simulink model "asbhl20_GuidanceApp"  (R2016b)
settings: Solver=FixedStepDiscrete  StartTime=0.0  StopTime=10.0  FixedStep=1/60  RelTol=1e-3
values from neighbouring files (symbols this model uses):
  Aimpoint = 500    [asbhl20_GuidanceAppData.mat]
  alpha0 = 0.114253174362    [asbhl20_GuidanceAppData.mat]
  fitdata =     [asbhl20_GuidanceAppData.mat]
  glideslope_offset = 20    [asbhl20_GuidanceAppData.mat]
  heading0 = 117    [asbhl20_GuidanceAppData.mat]
  hglide = [2 2.4375 2.875 3.3125 3.75 4.1875 4.625 5.0625 5.5 5.9375 6.375 6.8125 ... (668 elements, 668x1)]    [asbhl20_GuidanceAppData.mat]
  Xglide = [-675 -650 -625 -600 -575 -550 -525 -500 -475 -450 -425 -400 ... (668 elements, 668x1)]    [asbhl20_GuidanceAppData.mat]
undefined symbols (not defined in the file or in its folder): DiscIntNeverNeededParam, Earth, Tc, WGS84
libraries: asbhl20scdexblks x4, simulink x2, aerolibtransform2 x1, aerolibobsolete x1, aerolibconvert2 x1
Description:
  | HL-20 guidance control system module
settings Model: FPTRunName=Active  ExtModeAutoUpdateStatusClock=off  Creator=The MathWorks, Inc.  LastModifiedBy=The MathWorks, Inc.
settings DataIOCC: SaveFormat=Array  SaveOutput=off  SaveTime=off
settings OptimizationCC: BlockReduction=off  DefaultParameterBehavior=Inlined  OptimizeBlockIOStorage=off  BufferReuse=off  GlobalBufferReuse=off  ExpressionFolding=off  ExpressionDepthLimit=2147483647  LocalBlockOutputs=off  InitFltsAndDblsToZero=on  LifeSpan=inf
settings DebuggingCC: AlgebraicLoopMsg=none  UnderspecifiedInitializationDetection=Classic  MultiTaskCondExecSysMsg=none  FcnCallInpInsideContextMsg=warning  UnconnectedInputMsg=none  UnconnectedOutputMsg=none  UnconnectedLineMsg=none  UniqueDataStoreMsg=error  AllowSymbolicDim=off  StateNameClashWarn=warning  StrictBusMsg=ErrorOnBusTreatedAsVector  SFUnexpectedBacktrackingDiag=warning  SFNoUnconditionalDefaultTransitionDiag=warning  SFExecutionAtInitializationDiag=none
settings HardwareCC: ProdBitPerPointer=32  ProdBitPerSizeT=32  ProdBitPerPtrDiffT=32  ProdLargestAtomicFloat=None  ProdIntDivRoundTo=Undefined  ProdEndianess=Unspecified  ProdWordSize=32  ProdHWDeviceType=32-bit Generic
settings ModelReferenceCC: UpdateModelReferenceTargets=AssumeUpToDate  CheckModelReferenceTargetMessage=none  ModelReferencePassRootInputsByReference=off  PropagateSignalLabelsOutOfModel=off
settings CodeAppCC: MaxIdLength=63
settings GRTTargetCC: TargetLangStandard=C89/C90 (ANSI)  GeneratePreprocessorConditionals=Disable all  CombineOutputUpdateFcns=off  GRTInterface=on
settings ConfigComp: CovMetricSettings=dw  CovHtmlReporting=on  CovSaveCumulativeToWorkspaceVar=on  CovSaveSingleToWorkspaceVar=on  CovExternalEMLEnable=off  CovSFcnEnable=off

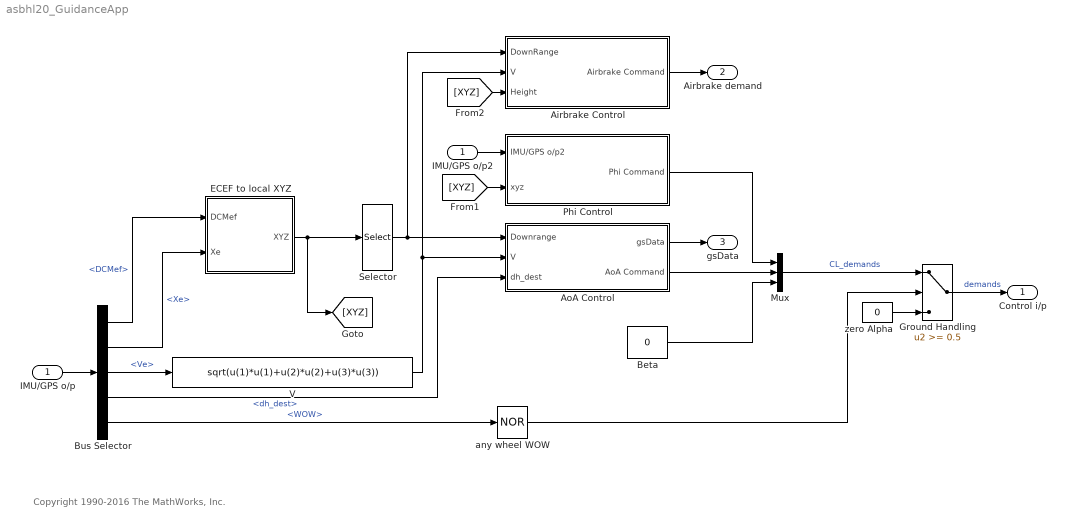
== system asbhl20_GuidanceApp ==
  note: Copyright 1990-2016 The MathWorks, Inc.
  IMU/GPS o/p : Inport  OutDataTypeStr=Bus: GuidanceBus
  Airbrake Control : Subsystem
  AoA Control : Subsystem
  Beta : Constant  Value=0  OutDataTypeStr=float('double')  SampleTime=Tc
  Bus Selector : BusSelector  OutputSignals=DCMef,Xe,Ve,dh_dest,WOW
  ECEF to local XYZ : Subsystem
  Ground Handling : Switch  Threshold=0.5  SaturateOnIntegerOverflow=on  InputSameDT=on
  IMU/GPS o/p2 : InportShadow  OutDataTypeStr=Bus: GuidanceBus
  Mux : Mux  Inputs=3
  Phi Control : Subsystem
  Selector : Selector  InputPortWidth=3  IndexOptions=Index vector (dialog)  Indices=1  OutputSizes=1
  V : Fcn  Expr=sqrt(u(1)*u(1)+u(2)*u(2)+u(3)*u(3))
  any wheel WOW : Logic  Operator=NOR  Inputs=1  IconShape=distinctive  AllPortsSameDT=off  OutDataTypeStr=boolean
  zero Alpha : Constant  Value=0  OutDataTypeStr=float('double')  SampleTime=Tc
  Control i/p : Outport
  Airbrake demand : Outport  Port=2
  gsData : Outport  Port=3  OutDataTypeStr=Bus: gsDataBus
  wires:
  Bus Selector/5 -> any wheel WOW/1  "<WOW>"
  any wheel WOW/1 -> Ground Handling/2
  Ground Handling/1 -> Control i/p/1  "demands"
  V/1 -> Airbrake Control/2(V), AoA Control/2(V)
  Mux/1 -> Ground Handling/1  "CL_demands"
  Bus Selector/2 -> ECEF to local XYZ/2(Xe)  "<Xe>"
  Bus Selector/3 -> V/1  "<Ve>"
  IMU/GPS o/p/1 -> Bus Selector/1
  Bus Selector/1 -> ECEF to local XYZ/1(DCMef)  "<DCMef>"
  ECEF to local XYZ/1(XYZ) -> [XYZ], Selector/1
  Selector/1 -> Airbrake Control/1(DownRange), AoA Control/1(Downrange)
  Phi Control/1(Phi Command) -> Mux/1
  IMU/GPS o/p2/1 -> Phi Control/1(IMU/GPS o/p2)
  zero Alpha/1 -> Ground Handling/3
  [XYZ] -> Phi Control/2(xyz)
  [XYZ] -> Airbrake Control/3(Height)
  Airbrake Control/1(Airbrake Command) -> Airbrake demand/1
  AoA Control/1(gsData) -> gsData/1
  AoA Control/2(AoA Command) -> Mux/2
  Bus Selector/4 -> AoA Control/3(dh_dest)  "<dh_dest>"
  Beta/1 -> Mux/3

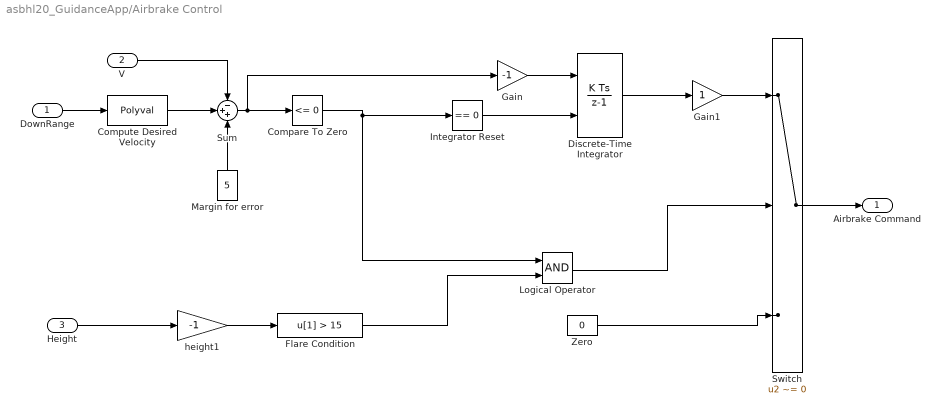
== system asbhl20_GuidanceApp/Airbrake Control ==
  DownRange : Inport
  V : Inport  Port=2
  Height : Inport  Port=3
  Compare To Zero : simulink/Logic and Bit Operations/Compare To Zero  relop=<=  OutDataTypeStr=uint8  ZeroCross=off
  Compute Desired Velocity : Polyval  Coefs=fitdata.coeff
  Discrete-Time Integrator : DiscreteIntegrator  ExternalReset=level  InitialConditionSetting=State (most efficient)  SampleTime=Tc  LimitOutput=on  UpperSaturationLimit=50  LowerSaturationLimit=-50  ICPrevOutput=DiscIntNeverNeededParam  ICPrevScaledInput=DiscIntNeverNeededParam
  Flare Condition : Fcn  Expr=u[1] > 15
  Gain : Gain  Gain=-1
  Gain1 : Gain
  Integrator Reset : simulink/Logic and Bit Operations/Compare To Zero  relop===  OutDataTypeStr=uint8  ZeroCross=off
  Logical Operator : Logic  AllPortsSameDT=off  OutDataTypeStr=boolean
  Margin for error : Constant  Value=5  OutDataTypeStr=float('double')  SampleTime=Tc
  Sum : Sum  Inputs=-++
  Switch : Switch  Criteria=u2 ~= 0
  Zero : Constant  Value=0  OutDataTypeStr=float('double')  SampleTime=Tc
  height1 : Gain  Gain=-1  SaturateOnIntegerOverflow=on  OutDataTypeStr=Inherit: Same as input  ParamDataTypeStr=Inherit: Same as input
  Airbrake Command : Outport
  wires:
  V/1 -> Sum/1
  Margin for error/1 -> Sum/3
  Gain1/1 -> Switch/1
  Logical Operator/1 -> Switch/2
  Flare Condition/1 -> Logical Operator/2
  height1/1 -> Flare Condition/1
  Height/1 -> height1/1
  Switch/1 -> Airbrake Command/1
  Zero/1 -> Switch/3
  Integrator Reset/1 -> Discrete-Time Integrator/2
  Discrete-Time Integrator/1 -> Gain1/1
  Gain/1 -> Discrete-Time Integrator/1
  Compare To Zero/1 -> Logical Operator/1, Integrator Reset/1
  Compute Desired Velocity/1 -> Sum/2
  Sum/1 -> Gain/1, Compare To Zero/1
  DownRange/1 -> Compute Desired Velocity/1

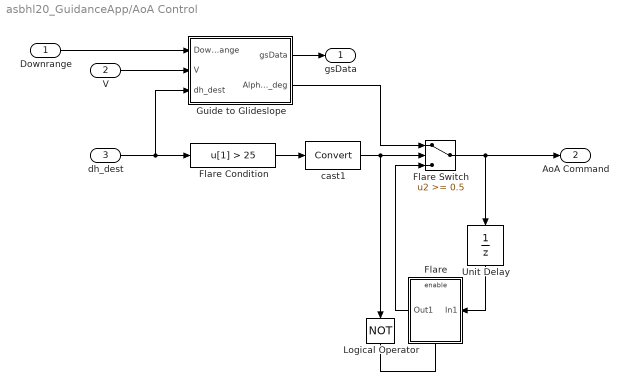
== system asbhl20_GuidanceApp/AoA Control ==
  Downrange : Inport
  V : Inport  Port=2
  dh_dest : Inport  Port=3
  Flare : Subsystem  TreatAsAtomicUnit=on
  Flare Condition : Fcn  Expr=u[1] > 25
  Flare Switch : Switch  Threshold=0.5  SaturateOnIntegerOverflow=on  InputSameDT=on
  Guide to Glideslope : Subsystem
  Logical Operator : Logic  Operator=NOT  IconShape=distinctive
  Unit Delay : UnitDelay  SampleTime=4*Tc
  cast1 : DataTypeConversion  SaturateOnIntegerOverflow=on  RndMeth=Zero
  gsData : Outport  OutDataTypeStr=Bus: gsDataBus
  AoA Command : Outport  Port=2
  wires:
  Guide to Glideslope/1(gsData) -> gsData/1
  Guide to Glideslope/2(AlphaD_deg) -> Flare Switch/1
  Logical Operator/1 -> Flare/Enable
  Flare/1(Out1) -> Flare Switch/3
  Flare Switch/1 -> Unit Delay/1, AoA Command/1
  Flare Condition/1 -> cast1/1
  cast1/1 -> Logical Operator/1, Flare Switch/2
  Unit Delay/1 -> Flare/1(In1)
  dh_dest/1 -> Flare Condition/1, Guide to Glideslope/3(dh_dest)
  Downrange/1 -> Guide to Glideslope/1(Downrange)
  V/1 -> Guide to Glideslope/2(V)

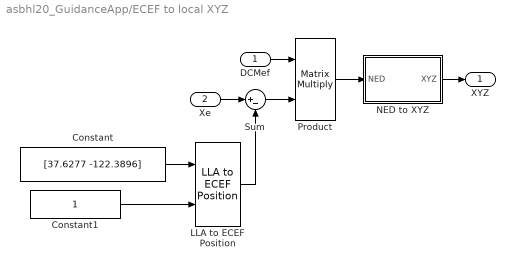
== system asbhl20_GuidanceApp/ECEF to local XYZ ==
  DCMef : Inport
  Xe : Inport  Port=2
  Constant : Constant  Value=[37.6277 -122.3896]
  Constant1 : Constant
  LLA to ECEF Position : aerolibtransform2/LLA to ECEF Position  units=Metric (MKS)  ptype=Earth (WGS84)  F=1/298.257223563  R=6378137
  NED to XYZ : Subsystem
  Product : Product  Multiplication=Matrix(*)  RndMeth=Zero
  Sum : Sum  Inputs=|+-
  XYZ : Outport
  wires:
  Sum/1 -> Product/2
  Constant1/1 -> LLA to ECEF Position/2
  Constant/1 -> LLA to ECEF Position/1
  LLA to ECEF Position/1 -> Sum/2
  Product/1 -> NED to XYZ/1(NED)
  DCMef/1 -> Product/1
  NED to XYZ/1(XYZ) -> XYZ/1
  Xe/1 -> Sum/1

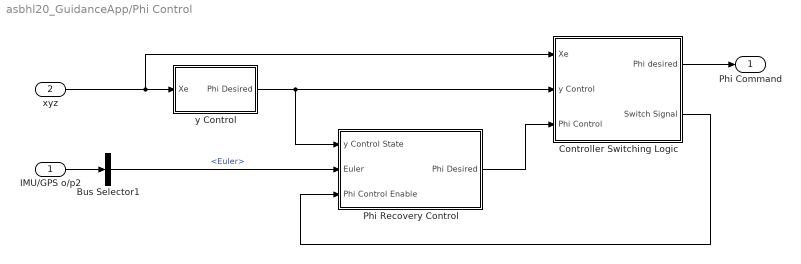
== system asbhl20_GuidanceApp/Phi Control ==
  IMU/GPS o/p2 : Inport
  xyz : Inport  Port=2
  Bus Selector1 : BusSelector  OutputSignals=Euler
  Controller Switching Logic : Subsystem
  Phi Recovery Control : Subsystem
  y Control : Subsystem
  Phi Command : Outport
  wires:
  y Control/1(Phi Desired) -> Phi Recovery Control/1(y Control State), Controller Switching Logic/2(y Control)
  Phi Recovery Control/1(Phi Desired) -> Controller Switching Logic/3(Phi Control)
  Controller Switching Logic/2(Switch Signal) -> Phi Recovery Control/3(Phi Control Enable)
  IMU/GPS o/p2/1 -> Bus Selector1/1
  Controller Switching Logic/1(Phi desired) -> Phi Command/1
  Bus Selector1/1 -> Phi Recovery Control/2(Euler)  "<Euler>"
  xyz/1 -> y Control/1(Xe), Controller Switching Logic/1(Xe)

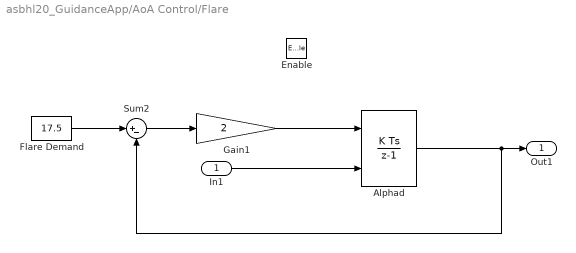
== system asbhl20_GuidanceApp/AoA Control/Flare ==
  In1 : Inport  SampleTime=Tc
  Enable : EnablePort  StatesWhenEnabling=reset
  Alphad : DiscreteIntegrator  InitialConditionSource=external  SampleTime=Tc  LimitOutput=on  UpperSaturationLimit=35  LowerSaturationLimit=-10  ICPrevOutput=DiscIntNeverNeededParam  ICPrevScaledInput=DiscIntNeverNeededParam
  Flare Demand : Constant  Value=17.5  OutDataTypeStr=float('double')
  Gain1 : Gain  Gain=2  SaturateOnIntegerOverflow=on  OutDataTypeStr=Inherit: Same as input  ParamDataTypeStr=Inherit: Same as input
  Sum2 : Sum  Inputs=|+-  SaturateOnIntegerOverflow=on  InputSameDT=on  OutDataTypeStr=Inherit: Same as first input
  Out1 : Outport
  wires:
  Alphad/1 -> Out1/1, Sum2/2
  Gain1/1 -> Alphad/1
  Sum2/1 -> Gain1/1
  Flare Demand/1 -> Sum2/1
  In1/1 -> Alphad/2

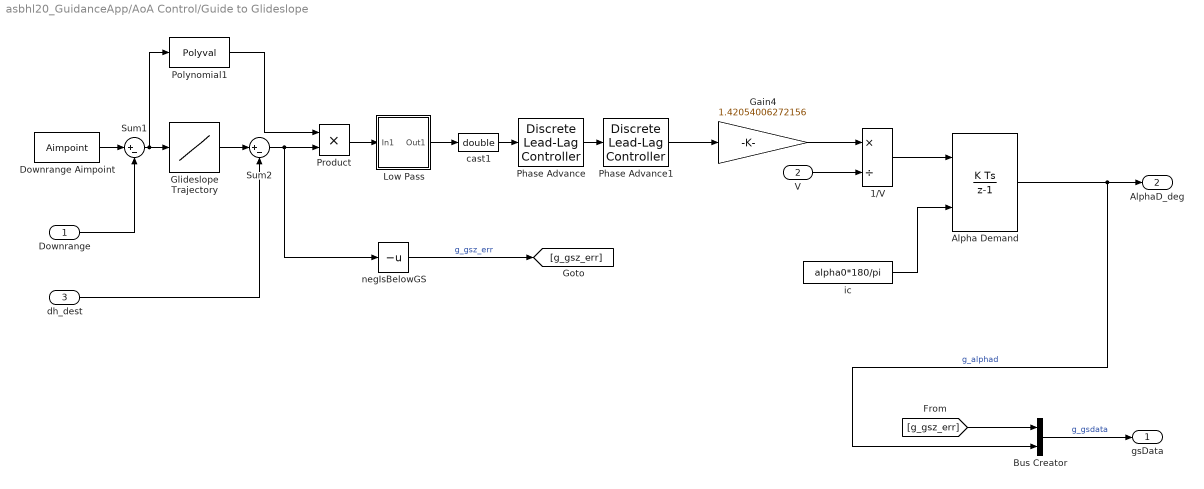
== system asbhl20_GuidanceApp/AoA Control/Guide to Glideslope ==
  Downrange : Inport
  V : Inport  Port=2
  dh_dest : Inport  Port=3
  1/V : Product  Inputs=*/  SaturateOnIntegerOverflow=on  InputSameDT=on  OutDataTypeStr=Inherit: Same as first input
  Alpha Demand : DiscreteIntegrator  InitialConditionSource=external  SampleTime=Tc  LimitOutput=on  UpperSaturationLimit=15  LowerSaturationLimit=0  ICPrevOutput=DiscIntNeverNeededParam  ICPrevScaledInput=DiscIntNeverNeededParam
  Bus Creator : BusCreator  Inputs=2  OutDataTypeStr=Bus: gsDataBus
  Downrange Aimpoint : Constant  Value=Aimpoint  OutDataTypeStr=float('double')
  Gain4 : Gain  Gain=1.42054006272156  SaturateOnIntegerOverflow=on  OutDataTypeStr=Inherit: Same as input  ParamDataTypeStr=Inherit: Same as input
  Glideslope Trajectory : Lookup_n-D  NumberOfTableDimensions=1  BreakpointsForDimension1=Xglide  Table=hglide+glideslope_offset  SaturateOnIntegerOverflow=on
  Low Pass : Subsystem
  Phase Advance : asbhl20scdexblks/Discrete Lead-Lag Controller  Zero=0.0620701951848126  Pole=16.8176549917091  Ts=Tc
  Phase Advance1 : asbhl20scdexblks/Discrete Lead-Lag Controller  Zero=0.286368115972358  Pole=16.8102119520749  Ts=Tc
  Polynomial1 : Polyval  Coefs=[-1/9249.5 1]
  Product : Product  RndMeth=Zero
  Sum1 : Sum  Inputs=|+-  SaturateOnIntegerOverflow=on  InputSameDT=on  OutDataTypeStr=Inherit: Same as first input
  Sum2 : Sum  Inputs=|+-  SaturateOnIntegerOverflow=on  InputSameDT=on  OutDataTypeStr=Inherit: Same as first input
  cast1 : DataTypeConversion  OutDataTypeStr=double
  ic : Constant  Value=alpha0*180/pi  OutDataTypeStr=float('double')
  negIsBelowGS : UnaryMinus
  gsData : Outport
  AlphaD_deg : Outport  Port=2
  wires:
  negIsBelowGS/1 -> [g_gsz_err]  "g_gsz_err"
  [g_gsz_err] -> Bus Creator/1
  Bus Creator/1 -> gsData/1  "g_gsdata"
  Downrange/1 -> Sum1/2
  dh_dest/1 -> Sum2/2
  V/1 -> 1/V/2
  1/V/1 -> Alpha Demand/1
  Gain4/1 -> 1/V/1
  Sum2/1 -> negIsBelowGS/1, Product/2
  Glideslope Trajectory/1 -> Sum2/1
  Sum1/1 -> Polynomial1/1, Glideslope Trajectory/1
  Downrange Aimpoint/1 -> Sum1/1
  ic/1 -> Alpha Demand/2
  Low Pass/1(Out1) -> cast1/1
  Phase Advance/1 -> Phase Advance1/1
  Phase Advance1/1 -> Gain4/1
  cast1/1 -> Phase Advance/1
  Polynomial1/1 -> Product/1
  Product/1 -> Low Pass/1(In1)
  Alpha Demand/1 -> Bus Creator/2, AlphaD_deg/1  "g_alphad"

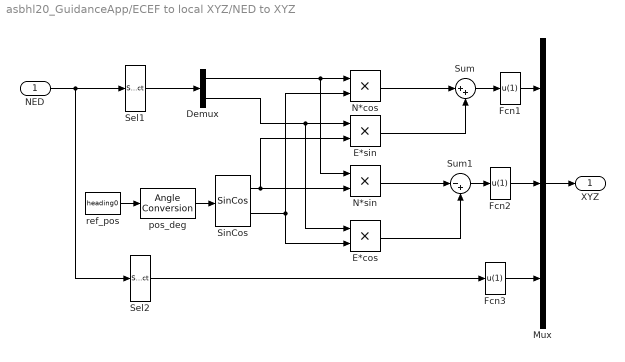
== system asbhl20_GuidanceApp/ECEF to local XYZ/NED to XYZ ==
  NED : Inport
  Demux : Demux  Outputs=2
  E*cos : Product  RndMeth=Zero
  E*sin : Product  RndMeth=Zero
  Fcn1 : Fcn  Expr=u(1)
  Fcn2 : Fcn  Expr=u(1)
  Fcn3 : Fcn  Expr=u(1)
  Mux : Mux  Inputs=3
  N*cos : Product  RndMeth=Zero
  N*sin : Product  RndMeth=Zero
  Sel1 : Selector  InputPortWidth=3  IndexOptions=Index vector (dialog)  Indices=[1,2]  OutputSizes=1
  Sel2 : Selector  InputPortWidth=3  IndexOptions=Index vector (dialog)  Indices=3  OutputSizes=1
  SinCos : aerolibobsolete/SinCos
  Sum : Sum  Inputs=|++
  Sum1 : Sum  Inputs=|-+
  pos_deg : aerolibconvert2/Angle Conversion  IU=deg  OU=rad
  ref_pos : Constant  Value=heading0
  XYZ : Outport
  wires:
  Sel2/1 -> Fcn3/1
  Sel1/1 -> Demux/1
  Mux/1 -> XYZ/1
  pos_deg/1 -> SinCos/1
  Demux/2 -> E*cos/1, E*sin/1
  Sum1/1 -> Fcn2/1
  E*cos/1 -> Sum1/2
  N*sin/1 -> Sum1/1
  Sum/1 -> Fcn1/1
  E*sin/1 -> Sum/2
  SinCos/1 -> N*sin/2, E*sin/2
  N*cos/1 -> Sum/1
  SinCos/2 -> E*cos/2, N*cos/2
  Demux/1 -> N*sin/1, N*cos/1
  NED/1 -> Sel2/1, Sel1/1
  ref_pos/1 -> pos_deg/1
  Fcn1/1 -> Mux/1
  Fcn2/1 -> Mux/2
  Fcn3/1 -> Mux/3

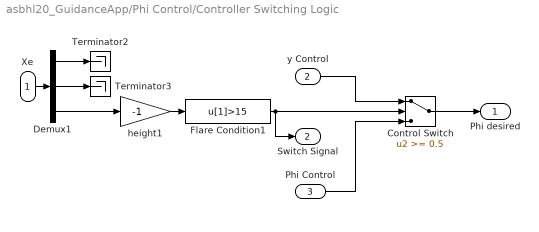
== system asbhl20_GuidanceApp/Phi Control/Controller Switching Logic ==
  Xe : Inport
  y Control : Inport  Port=2
  Phi Control : Inport  Port=3
  Control Switch : Switch  Threshold=0.5  SaturateOnIntegerOverflow=on  InputSameDT=on
  Demux1 : Demux  Outputs=3
  Flare Condition1 : Fcn  Expr=u[1]>15
  Terminator2 : Terminator
  Terminator3 : Terminator
  height1 : Gain  Gain=-1  SaturateOnIntegerOverflow=on  OutDataTypeStr=Inherit: Same as input  ParamDataTypeStr=Inherit: Same as input
  Phi desired : Outport
  Switch Signal : Outport  Port=2
  wires:
  Control Switch/1 -> Phi desired/1
  Phi Control/1 -> Control Switch/3
  y Control/1 -> Control Switch/1
  Demux1/2 -> Terminator3/1
  Flare Condition1/1 -> Switch Signal/1, Control Switch/2
  Xe/1 -> Demux1/1
  Demux1/3 -> height1/1
  Demux1/1 -> Terminator2/1
  height1/1 -> Flare Condition1/1

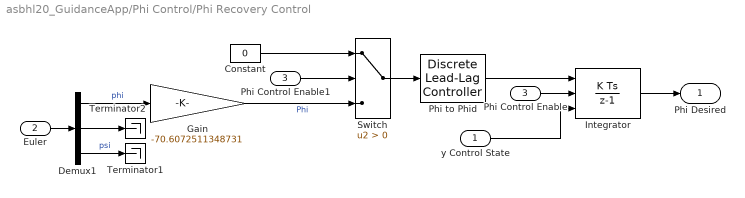
== system asbhl20_GuidanceApp/Phi Control/Phi Recovery Control ==
  y Control State : Inport
  Euler : Inport  Port=2
  Phi Control Enable : Inport  Port=3
  Constant : Constant  Value=0
  Demux1 : Demux  Outputs=3
  Gain : Gain  Gain=-70.6072511348731
  Integrator : DiscreteIntegrator  ExternalReset=level  InitialConditionSource=external  SampleTime=Tc  LimitOutput=on  UpperSaturationLimit=20  LowerSaturationLimit=-20  ICPrevOutput=DiscIntNeverNeededParam  ICPrevScaledInput=DiscIntNeverNeededParam  mask(DiscretizedDiscreteIntegrator){}
      mask init:
      | %zoh
  Phi Control Enable1 : InportShadow  Port=3
  Phi to Phid : asbhl20scdexblks/Discrete Lead-Lag Controller  Zero=15  Pole=50  Ts=Tc
  Switch : Switch  Criteria=u2 > Threshold
  Terminator1 : Terminator
  Terminator2 : Terminator
  Phi Desired : Outport
  wires:
  Constant/1 -> Switch/1
  Phi Control Enable1/1 -> Switch/2
  Gain/1 -> Switch/3  "Phi"
  Switch/1 -> Phi to Phid/1
  Demux1/3 -> Terminator1/1  "psi"
  Euler/1 -> Demux1/1
  y Control State/1 -> Integrator/3
  Phi Control Enable/1 -> Integrator/2
  Integrator/1 -> Phi Desired/1
  Phi to Phid/1 -> Integrator/1
  Demux1/1 -> Gain/1  "phi"
  Demux1/2 -> Terminator2/1

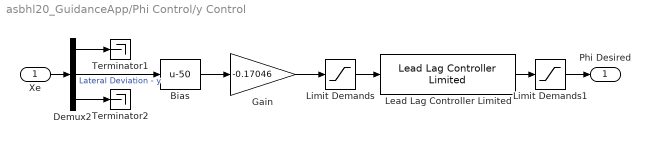
== system asbhl20_GuidanceApp/Phi Control/y Control ==
  Xe : Inport
  Bias : Bias  Bias=-50
  Demux2 : Demux  Outputs=3
  Gain : Gain  Gain=-0.17046
  Lead Lag Controller Limited : asbhl20scdexblks/Lead Lag Controller Limited  ZF=0.0400436516896399  PF=15.0000560854201  Ts=Tc  lower_limit=-498.1  upper_limit=498.1
  Limit Demands : Saturate  UpperLimit=20  LowerLimit=-20
  Limit Demands1 : Saturate  UpperLimit=20  LowerLimit=-20
  Terminator1 : Terminator
  Terminator2 : Terminator
  Phi Desired : Outport
  wires:
  Lead Lag Controller Limited/1 -> Limit Demands1/1
  Xe/1 -> Demux2/1
  Demux2/3 -> Terminator2/1
  Demux2/2 -> Bias/1  "Lateral Deviation - y"
  Demux2/1 -> Terminator1/1
  Gain/1 -> Limit Demands/1
  Bias/1 -> Gain/1
  Limit Demands/1 -> Lead Lag Controller Limited/1
  Limit Demands1/1 -> Phi Desired/1

== system asbhl20_GuidanceApp/AoA Control/Guide to Glideslope/Low Pass ==
  In1 : Inport
  Omega : Gain  Gain=2  SaturateOnIntegerOverflow=on  OutDataTypeStr=Inherit: Same as input  ParamDataTypeStr=Inherit: Same as input
  Sum3 : Sum  Inputs=|+-  SaturateOnIntegerOverflow=on  InputSameDT=on  OutDataTypeStr=Inherit: Same as first input
  filterState : Subsystem  mask(DiscretizedIntegrator){integratormethod=Forward Euler, externalreset=none, initialconditionsource=external, limitoutput=on, uppersaturationlimit=-inf, lowersaturationlimit=inf, showsaturationport=off, showstateport=off, absolutetolerance=auto, enablezerocrossingdetection=on, SampleTime=Tc}
      mask prompts: integratormethod "Integrator method:"; externalreset "External reset:"; initialconditionsource "Initial condition source"; limitoutput "Limit output"; uppersaturationlimit "Upper saturation limit:"; lowersaturationlimit "Lower saturation limit:"; showsaturationport "Show saturation port"; showstateport "Show state port"; absolutetolerance "Absolute tolerance:"; enablezerocrossingdetection "Enable zero crossing detection"; SampleTime "Sample time:"
      mask help: Swap between continuous integrator and discrete integrator based on sample time.
      mask init:
      | blk = gcb;
      | st=SampleTime; if length(st)>1, st=SampleTime(1); end
      | 
      | iname = [blk, '/Integrator'];
      | if(st==0),
      | 	method = '';
      | 	if ~strcmp(get_param(iname,'BlockType'),'Integrator'),
      |         mv = get_param(gcb,'maskvalues');
      | 		abstolStr = mv{9};
      | 		pos = get_param(iname, 'Position');
      | 		newtype = 'built-in/Integrator';
      | 		delete_block(iname);
      | 		add_block(newtype, iname, 'Position', pos, 'InitialConditionSource', 'external', 'AbsoluteTolerance', '1');
      | 	end
      | else
      |     mv = get_param(gcb,'maskvalues');
      | 	method = mv{1};
      | 	if strcmp(get_param(iname,'BlockType'),'Integrator'),
      | 		pos = get_param(iname, 'Position');
      | 		newtype = 'built-in/DiscreteIntegrator';
      | 		delete_block(iname);
      | 		add_block(newtype, iname, 'Position', pos, 'IntegratorMethod', method, 'InitialConditionSource', 'external', 'SampleTime', 'SampleTime');
      | 	else
      | 		set_param(iname, 'IntegratorMethod', method);
      | 	end
      | end
      mask TypeOptions integratormethod: Forward Euler | Backward Euler | Trapezoidal
      mask TypeOptions externalreset: none | rising | falling | either | level
      mask TypeOptions initialconditionsource: internal | external
      mask Display:
      | dpoly(1, [1,0], 's')
      | text( 0.5, 1.0, method, 'verticalAlignment','top')
      | port_label('input', 2, 'Xo')
  Out1 : Outport
  wires:
  Omega/1 -> filterState/1(In1)
  Sum3/1 -> Omega/1
  filterState/1(Out1) -> Sum3/2, Out1/1
  In1/1 -> filterState/2(In2), Sum3/1

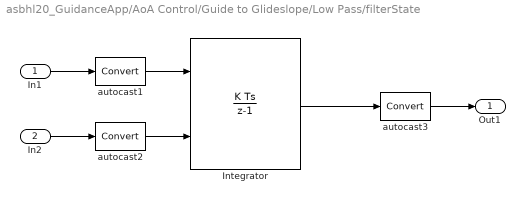
== system asbhl20_GuidanceApp/AoA Control/Guide to Glideslope/Low Pass/filterState ==
  In1 : Inport
  In2 : Inport  Port=2
  Integrator : DiscreteIntegrator  InitialConditionSource=external  SampleTime=SampleTime  ICPrevOutput=DiscIntNeverNeededParam  ICPrevScaledInput=DiscIntNeverNeededParam
  autocast1 : DataTypeConversion  SaturateOnIntegerOverflow=on  RndMeth=Zero
  autocast2 : DataTypeConversion  SaturateOnIntegerOverflow=on  RndMeth=Zero
  autocast3 : DataTypeConversion  SaturateOnIntegerOverflow=on  RndMeth=Zero
  Out1 : Outport
  wires:
  In2/1 -> autocast2/1
  autocast2/1 -> Integrator/2
  Integrator/1 -> autocast3/1
  In1/1 -> autocast1/1
  autocast1/1 -> Integrator/1
  autocast3/1 -> Out1/1
